simulink model "embedded_with_for_and_eps"  (Simulink 7.6)
settings: Solver=FixedStepDiscrete  StartTime=0.0  StopTime=10.0  FixedStep=1  RelTol=1e-3
PreLoadFcn:
  | ControlParameters
settings Model: Creator=Harmon S. Nine  LastModifiedBy=c2wt
settings DataIOCC: SaveFormat=Structure
settings DebuggingCC: StrictBusMsg=Warning
settings SFSimCC: SimParseCustomCode=off

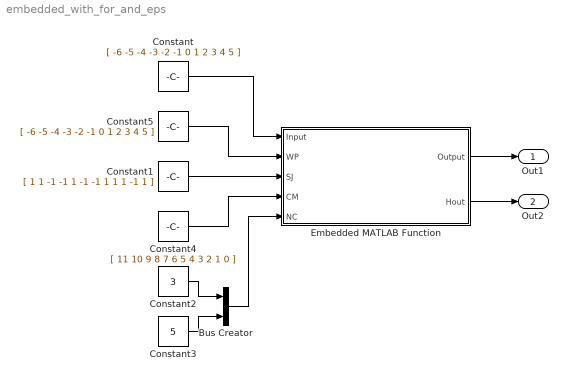
== system embedded_with_for_and_eps ==
  Bus Creator : BusCreator  Inputs=2  OutDataTypeStr=Bus: ControlParameters  NonVirtualBus=on
  Constant : Constant  Value=[ -6 -5 -4 -3 -2 -1 0 1 2 3 4 5 ]  VectorParams1D=off
  Constant1 : Constant  Value=[ 1 1 -1 -1 1 -1 -1 1 1 1 -1 1 ]  VectorParams1D=off
  Constant2 : Constant  Value=3  VectorParams1D=off  OutDataTypeStr=single
  Constant3 : Constant  Value=5  OutDataTypeStr=single
  Constant4 : Constant  Value=[ 11 10 9 8 7 6 5 4 3 2 1 0 ]  VectorParams1D=off
  Constant5 : Constant  Value=[ -6 -5 -4 -3 -2 -1 0 1 2 3 4 5 ]  VectorParams1D=off
  Embedded MATLAB Function : Stateflow chart  TreatAsAtomicUnit=on
  Out1 : Outport
  Out2 : Outport  Port=2
  wires:
  Embedded MATLAB Function/1(Output) -> Out1/1
  Constant/1 -> Embedded MATLAB Function/1(Input)
  Constant1/1 -> Embedded MATLAB Function/3(SJ)
  Embedded MATLAB Function/2(Hout) -> Out2/1
  Bus Creator/1 -> Embedded MATLAB Function/5(NC)
  Constant2/1 -> Bus Creator/1
  Constant3/1 -> Bus Creator/2
  Constant4/1 -> Embedded MATLAB Function/4(CM)
  Constant5/1 -> Embedded MATLAB Function/2(WP)

== matlab function Embedded MATLAB Function ==
  data: Output output double; Input input double; WP input double; SJ input double; CM input double; NC input double; Hout output double
function [ Output, Hout ] = fcn( Input, WP, SJ, CM, NC )
%#eml

eml.inline( 'never' );

% Output declarations
Output = zeros(12,1,'single');
Hout = zeros(12,1,'uint32');

for index=1:12
                
    % By default, assign the output to the input
    Output(index) = Input(index);
    
    if (SJ(index) > 0 && Input(index) < eps('single'))

        if (CM(index) == 3) 
            Hout(index) = 0;      
        elseif (WP(index) < NC.WPM)
            Output(index) = NC.TC;
            Hout(index) = 1;
        end
    end
    
end
